simulink model "validacao"  (R2018b)
settings: Solver=FixedStepAuto  StartTime=0.0  StopTime=5  FixedStep=0.01  RelTol=1e-3
values from neighbouring files (symbols this model uses):
  teste6 = [0 0 0 0 0 0 0 0 0 0 0 0 ... (1737 elements, 579x3)]    [identificacao.mat]
libraries: simulink x2
settings Model: Creator=lubuntu  LastModifiedBy=lubuntu

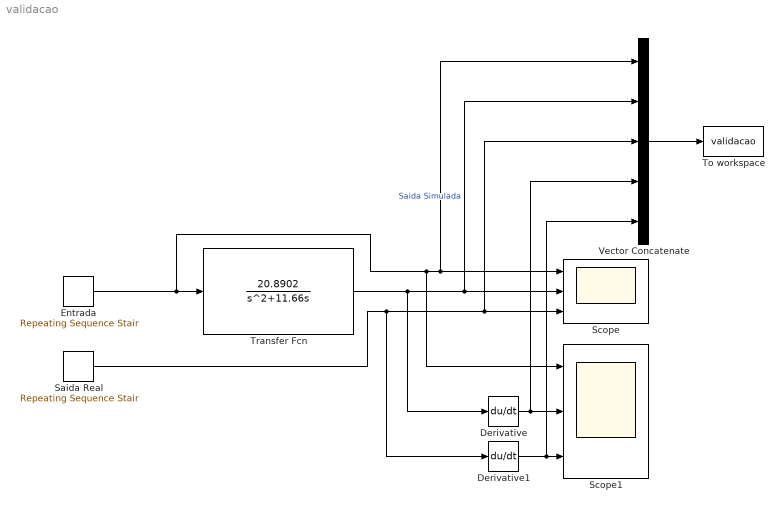
== system validacao ==
  Derivative : Derivative
  Derivative1 : Derivative
  Entrada : simulink/Sources/Repeating Sequence Stair  OutValues=teste6(:,1)  tsamp=0.01  OutMin=[]  OutMax=[]  OutDataTypeStr=double  OutputDataTypeScalingMode=double  OutDataType=fixdt(0,8)  ConRadixGroup=Best Precision: Vector-wise  OutScaling=2^-12
  Saida Real : simulink/Sources/Repeating Sequence Stair  OutValues=teste6(:,2)  tsamp=0.01  OutMin=[]  OutMax=[]  OutDataTypeStr=double  OutputDataTypeScalingMode=double  OutDataType=fixdt(0,8)  ConRadixGroup=Best Precision: Vector-wise  OutScaling=2^-12
  Scope : Scope  NumInputPorts=3
  Scope1 : Scope  NumInputPorts=3
  To workspace : ToWorkspace  VariableName=validacao  SaveFormat=Timeseries  SampleTime=-1
  Transfer Fcn : TransferFcn  Numerator=[ 20.8902 ]  Denominator=[1 11.66 0]
  Vector Concatenate : Concatenate  NumInputs=5
  wires:
  Entrada/1 -> Scope/1, Vector Concatenate/1, Scope1/1, Transfer Fcn/1
  Transfer Fcn/1 -> Scope/2, Vector Concatenate/2, Derivative/1  "Saida Simulada"
  Saida Real/1 -> Scope/3, Vector Concatenate/3, Derivative1/1
  Derivative1/1 -> Vector Concatenate/5, Scope1/3
  Derivative/1 -> Scope1/2, Vector Concatenate/4
  Vector Concatenate/1 -> To workspace/1
